simulink model "caravan_battery_model"  (R2023a)
settings: Solver=VariableStepAuto  StartTime=0.0  StopTime=10.0  RelTol=1e-3
undefined symbols (not defined in the file or in its folder): Ion, Lithium
libraries: spsControlledCurrentSourceLib x1, spsBatteryLib x1, eeGeneralControl x1, spspowerguiLib x1
settings Model: Creator=TJBakker  LastModifiedBy=sandu

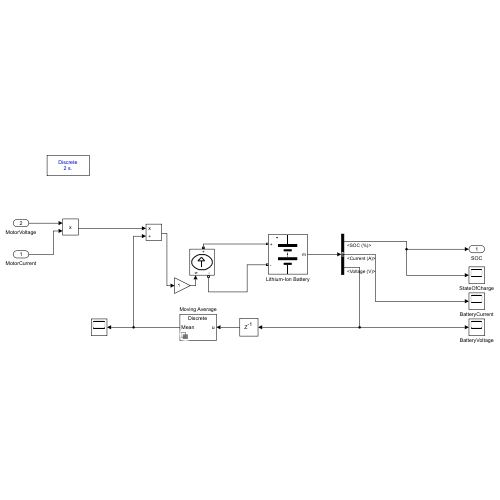
[thumbnail: Simulink's stored preview of the top-level diagram]
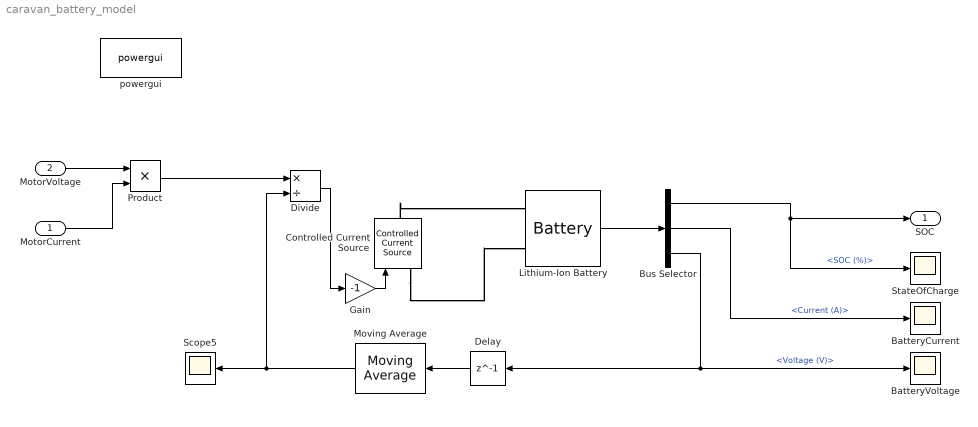
== system caravan_battery_model ==
  MotorCurrent : Inport
  MotorVoltage : Inport  Port=2
  BatteryCurrent : Scope
  BatteryVoltage : Scope
  Bus Selector : BusSelector  OutputSignals=SOC (%),Current (A),Voltage (V)
  Controlled Current Source : spsControlledCurrentSourceLib/Controlled Current Source  Initialize=on  Source_Type=AC  Amplitude=0  Phase=0  Frequency=0  Measurements=None
  Delay : Delay  DelayLength=1  InitialCondition=0
  Divide : Product  Inputs=*/
  Gain : Gain  Gain=-1
  Lithium-Ion Battery : spsBatteryLib/Battery  BatType=Lithium-Ion  ShowTempParam=off  ThermalPreset=no  ShowAgeParam=on  NomV=370  NomQ=300  SOC=100  Batt_Tr=0.1  PresetModel=on  MaxQ=300  MinV=277.5  FullV=430.6752  Dis_rate=130.4348  R=0.012333  Normal_OP=271.3043  expZone="[399.7428      14.73913]"  current=[1.2 0.6 0.3]  Units=Time  Tci=20  NomT=25  T2=0  MaxQ2=2.208  FullV2=3.45  Normal_OP2=2.8  expZone2="[3.22        0.23]"  Rca=0.6  ti=1000  Dp=0  Neq0=0  Tsim=1e6  Ta1=25  Qeol=5.4*0.9  Reol=0.013333*1.2  Char_age=[2.3478, 3]  Dis_age=[2.3478, 10]  N1=1500  N2=10500  N3=1000  N4=1400  Ta2=45  N5=950
      settings: LibrarySourceBlock=electricdrivelib/Extra Sources/Battery
  Moving Average : eeGeneralControl/Moving Average  VariantControl=Variant1  LabelModeActiveChoice=Discrete  f=0.01  x0=420  BufferSize=8192  Ts=-1
      settings: LibrarySourceBlock=ee_sl_lib/General Control/Moving Average
  Product : Product
  Scope5 : Scope
  StateOfCharge : Scope
  powergui : spspowerguiLib/powergui  Priority=1  SimulationMode=Discrete  SampleTime=2  frequency=60  Iterations=50  frequencyindice=0  Pbase=100e6  ErrMax=1e-4  UnitsV=kV  UnitsW=MW  buscounter=0  FunctionMessages=off  echomessages=off  EnableUseOfTLC=off  CurrentSourceSwitches=off  DisableSnubberDevices=off  DisableRonSwitches=off  DisableVfSwitches=off  DisplayEquations=off  AutomaticDiscreteSolvers=off  SolverType=Tustin/Backward Euler (TBE)  Interpol=off  ExternalGateDelay=off  methode=off  Ts=100  x0status=blocks  SPID=on  SwTol=0  HookPort=off  NonlinearTolerance=1e-4  nMaxIteration=100  ContinueOnMaxIteration=off  RestoreLinks=warning  ResistiveCurrentMeasurement=off  Frange=[0:2:500]  Ylog=off  Xlog=on  ShowGrid=off  save=off  variable=ZData  structure=0  ZoomFFT=off  StartTime=0.0  cycles=1  DisplayStyle=1  fundamental=60  FreqAxis=off  MaxFrequency=1000  frequencyindicesteady=1  RmsSteady=1  display=off
  SOC : Outport
  wires:
  Divide/1 -> Gain/1
  Product/1 -> Divide/1
  Moving Average/1 -> Divide/2, Scope5/1
  Bus Selector/1 -> SOC/1, StateOfCharge/1  "<SOC (%)>"
  Delay/1 -> Moving Average/1
  Bus Selector/2 -> BatteryCurrent/1  "<Current (A)>"
  Bus Selector/3 -> Delay/1, BatteryVoltage/1  "<Voltage (V)>"
  Gain/1 -> Controlled Current Source/1
  Lithium-Ion Battery/1 -> Bus Selector/1
  MotorVoltage/1 -> Product/1
  MotorCurrent/1 -> Product/2
  connections:
  Controlled Current Source/LConn1 -- Lithium-Ion Battery/LConn2
  Controlled Current Source/RConn1 -- Lithium-Ion Battery/LConn1
